simulink model "q5_model"  (R2020a)
settings: Solver=VariableStepAuto  StartTime=0.0  StopTime=10.0  RelTol=1e-3
settings Model: Creator=kiran  LastModifiedBy=kiran

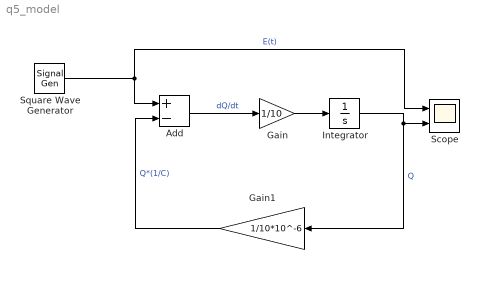
== system q5_model ==
  Add : Sum  Inputs=+-
  Gain : Gain  Gain=1/10
  Gain1 : Gain  Gain=1/10*10^-6
  Integrator : Integrator  InitialCondition=4
  Scope : Scope  NumInputPorts=2
  Square Wave Generator : SignalGenerator  WaveForm=square  Units=rad/sec
  wires:
  Square Wave Generator/1 -> Scope/1, Add/1  "E(t)"
  Gain1/1 -> Add/2  "Q*(1/C)"
  Add/1 -> Gain/1  "dQ/dt"
  Integrator/1 -> Scope/2, Gain1/1  "Q"
  Gain/1 -> Integrator/1
